simulink model "newzn"  (R2021a)
settings: Solver=VariableStepAuto  StartTime=0.0  StopTime=688000  RelTol=1e-3
values from neighbouring files (symbols this model uses):
  Ts = 0.5    [Distillation_Column_model_identification.m]    (also in Distillation_Column_model_variance.m; fourvary.m = 8)
libraries: cstblocks x2, dspsrcs4 x1
settings Model: Creator=dell  LastModifiedBy=dell
settings DataIOCC: LoadExternalInput=on

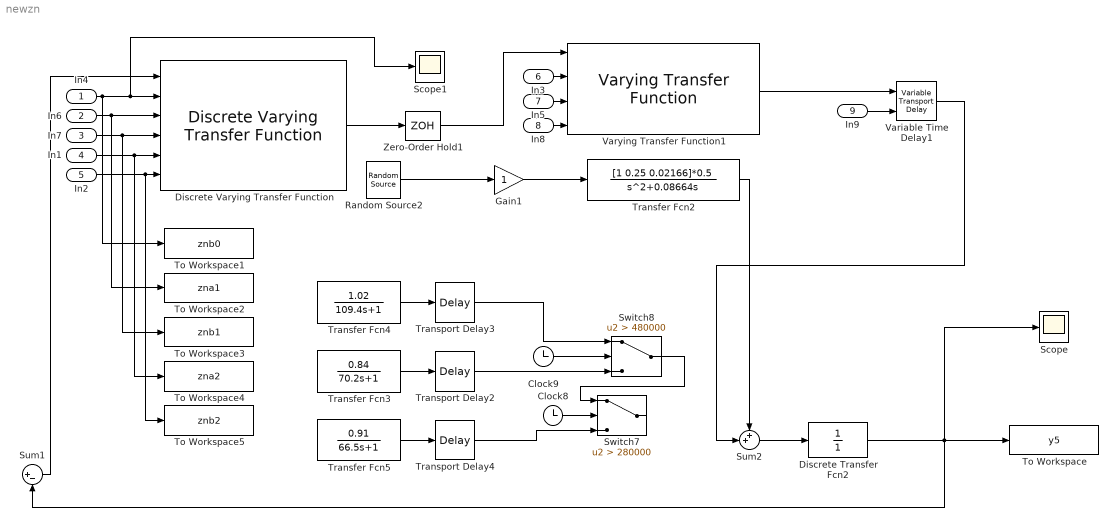
== system newzn ==
  In4 : Inport
  In6 : Inport  Port=2
  In7 : Inport  Port=3
  In1 : Inport  Port=4
  In2 : Inport  Port=5
  In3 : Inport  Port=6
  In5 : Inport  Port=7
  In8 : Inport  Port=8
  In9 : Inport  Port=9
  Clock8 : Clock
  Clock9 : Clock
  Discrete Transfer Fcn2 : DiscreteTransferFcn  Denominator=[1]  SampleTime=Ts
      mask Display: disp('sampler')
  Discrete Varying Transfer Function : cstblocks/Linear Parameter Varying/Discrete Varying Transfer Function  N=2  Ts=-1
      settings: SourceProductBaseCode=CT
  Gain1 : Gain
  Random Source2 : dspsrcs4/Random Source  SrcType=Gaussian  NormMethod=Ziggurat  CltLength=12  MinVal=-1  MaxVal=1  MeanVal=0  VarVal=1  RepMode=Specify seed  rawSeed=seed  IsInherit=off  SampMode=Continuous  SampTime=1  SampFrame=1  DataType=Double  OutComplex=Real  OutputFrames=off
  Scope : Scope
  Scope1 : Scope
  Sum1 : Sum  Inputs=|+-
  Sum2 : Sum  Inputs=++|
  Switch7 : Switch  Criteria=u2 > Threshold  Threshold=280000
  Switch8 : Switch  Criteria=u2 > Threshold  Threshold=480000
  To Workspace : ToWorkspace  VariableName=y5  SampleTime=Ts
  To Workspace1 : ToWorkspace  VariableName=znb0  SampleTime=Ts
  To Workspace2 : ToWorkspace  VariableName=zna1  SampleTime=Ts
  To Workspace3 : ToWorkspace  VariableName=znb1  SampleTime=Ts
  To Workspace4 : ToWorkspace  VariableName=zna2  SampleTime=Ts
  To Workspace5 : ToWorkspace  VariableName=znb2  SampleTime=Ts
  Transfer Fcn2 : TransferFcn  Numerator=[1 0.25 0.02166]*0.5  Denominator=[1 0.08664 0]
  Transfer Fcn3 : TransferFcn  Numerator=[0.84]  Denominator=[70.2 1]
  Transfer Fcn4 : TransferFcn  Numerator=[1.02]  Denominator=[109.4 1]
  Transfer Fcn5 : TransferFcn  Numerator=[0.91]  Denominator=[66.5 1]
  Transport Delay2 : TransportDelay  DelayTime=154
  Transport Delay3 : TransportDelay  DelayTime=157
  Transport Delay4 : TransportDelay  DelayTime=148
  Variable Time Delay1 : VariableTransportDelay  MaximumDelay=200
  Varying Transfer Function1 : cstblocks/Linear Parameter Varying/Varying Transfer Function  N=1
  Zero-Order Hold1 : ZeroOrderHold  SampleTime=Ts
  wires:
  Transfer Fcn2/1 -> Sum2/1
  Sum2/1 -> Discrete Transfer Fcn2/1
  Transport Delay3/1 -> Switch8/1
  Transfer Fcn4/1 -> Transport Delay3/1
  Transfer Fcn3/1 -> Transport Delay2/1
  Clock9/1 -> Switch8/2
  Clock8/1 -> Switch7/2
  Gain1/1 -> Transfer Fcn2/1
  Transfer Fcn5/1 -> Transport Delay4/1
  Transport Delay4/1 -> Switch7/3
  Random Source2/1 -> Gain1/1
  Switch8/1 -> Switch7/1
  Transport Delay2/1 -> Switch8/3
  Discrete Varying Transfer Function/1 -> Zero-Order Hold1/1
  Discrete Transfer Fcn2/1 -> Scope/1, Sum1/2, To Workspace/1
  In4/1 -> Scope1/1, Discrete Varying Transfer Function/2, To Workspace1/1
  In6/1 -> To Workspace2/1, Discrete Varying Transfer Function/3
  In7/1 -> To Workspace3/1, Discrete Varying Transfer Function/4
  In1/1 -> To Workspace4/1, Discrete Varying Transfer Function/5
  In2/1 -> To Workspace5/1, Discrete Varying Transfer Function/6
  Sum1/1 -> Discrete Varying Transfer Function/1
  Zero-Order Hold1/1 -> Varying Transfer Function1/1
  Varying Transfer Function1/1 -> Variable Time Delay1/1
  Variable Time Delay1/1 -> Sum2/2
  In9/1 -> Variable Time Delay1/2
  In8/1 -> Varying Transfer Function1/4
  In5/1 -> Varying Transfer Function1/3
  In3/1 -> Varying Transfer Function1/2
